simulink model "mixer"  (R2024b)
settings: configuration reference "simulation" (kept outside this file)
values from neighbouring files (symbols this model uses):
  fw_mixers =     [mixer_data.mat]
  mc_mixers =     [mixer_data.mat]
undefined symbols (not defined in the file or in its folder): MC_AIRMODE, MOT_SLEW_MAX, PWM_AUX_DIS1, PWM_AUX_DIS2, PWM_AUX_DIS3, PWM_AUX_DIS4, PWM_AUX_DIS5, PWM_AUX_DIS6, PWM_AUX_DIS7, PWM_AUX_DIS8, PWM_AUX_DISARM, PWM_AUX_FAIL1, PWM_AUX_FAIL2, PWM_AUX_FAIL3, PWM_AUX_FAIL4, PWM_AUX_FAIL5, PWM_AUX_FAIL6, PWM_AUX_FAIL7, PWM_AUX_FAIL8, PWM_AUX_MAX, PWM_AUX_MAX1, PWM_AUX_MAX2, PWM_AUX_MAX3, PWM_AUX_MAX4, PWM_AUX_MAX5, PWM_AUX_MAX6, PWM_AUX_MAX7, PWM_AUX_MAX8, PWM_AUX_MIN, PWM_AUX_MIN1, PWM_AUX_MIN2, PWM_AUX_MIN3, PWM_AUX_MIN4, PWM_AUX_MIN5, PWM_AUX_MIN6, PWM_AUX_REV1, PWM_AUX_REV2, PWM_AUX_REV3, PWM_AUX_REV4, PWM_AUX_REV5, PWM_AUX_REV6, PWM_AUX_REV7, PWM_AUX_REV8, PWM_AUX_TRIM1, PWM_AUX_TRIM2, PWM_AUX_TRIM3, PWM_AUX_TRIM4, PWM_AUX_TRIM5, PWM_AUX_TRIM6, PWM_AUX_TRIM7, PWM_AUX_TRIM8, PWM_MAIN_DIS1, PWM_MAIN_DIS2, PWM_MAIN_DIS3, PWM_MAIN_DIS4, PWM_MAIN_DIS5, PWM_MAIN_DIS6, PWM_MAIN_DIS7, PWM_MAIN_DIS8, PWM_MAIN_DISARM ... (+43)
libraries: simulink x4
settings Model: DataDictionary=nextpilot_datadict.sldd  Creator=CETCA  LastModifiedBy=93114
settings ConfigSetRef: SourceName=simulation

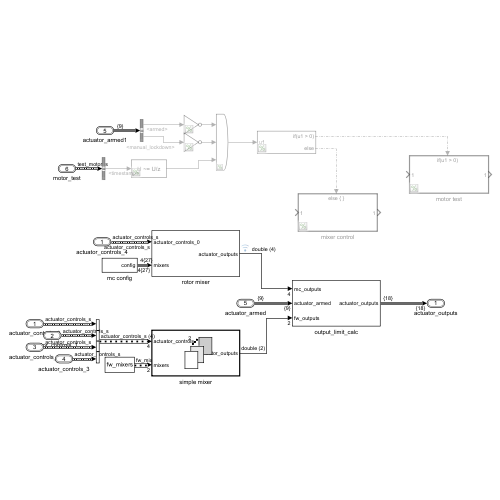
[thumbnail: Simulink's stored preview of the top-level diagram]
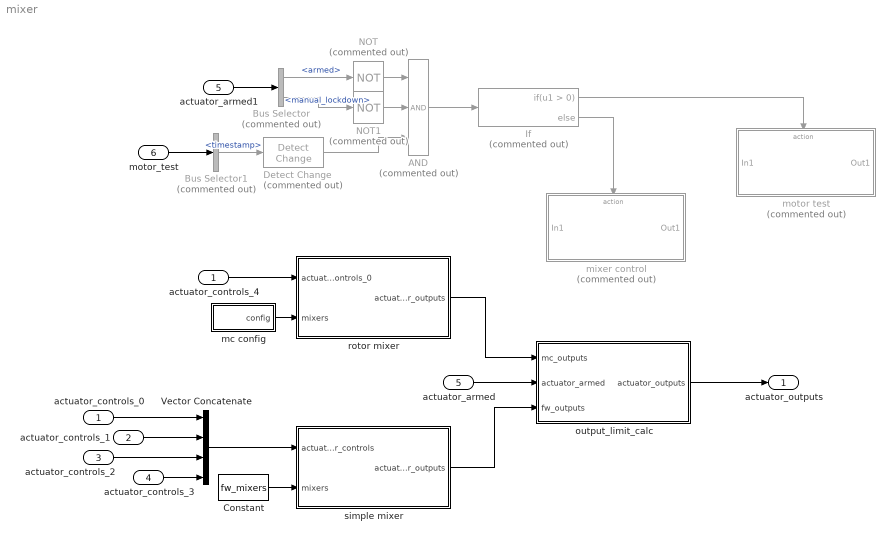
== system mixer ==
  actuator_controls_0 : Inport  OutDataTypeStr=Bus: actuator_controls_s  BusOutputAsStruct=on
  actuator_controls_1 : Inport  Port=2  OutDataTypeStr=Bus: actuator_controls_s  BusOutputAsStruct=on
  actuator_controls_2 : Inport  Port=3  OutDataTypeStr=Bus: actuator_controls_s  BusOutputAsStruct=on
  actuator_controls_3 : Inport  Port=4  OutDataTypeStr=Bus: actuator_controls_s  BusOutputAsStruct=on
  actuator_armed : Inport  Port=5  OutDataTypeStr=Bus: actuator_armed_s
  motor_test : Inport  Port=6  OutDataTypeStr=Bus: test_motor_s  BusOutputAsStruct=on
  AND : Logic  Commented=on  Inputs=3  IconShape=distinctive  AllPortsSameDT=off  OutDataTypeStr=boolean
  Bus Selector : BusSelector  Commented=on  OutputSignals=armed,manual_lockdown
  Bus Selector1 : BusSelector  Commented=on  OutputSignals=timestamp
  Constant : Constant  Value=fw_mixers  OutDataTypeStr=Bus: fw_mixer_s
  Detect Change : simulink/Logic and Bit Operations/Detect Change  Commented=on  vinit=0  OutDataTypeStr=boolean
  If : If  Commented=on
  NOT : Logic  Commented=on  Operator=NOT  IconShape=distinctive  AllPortsSameDT=off  OutDataTypeStr=boolean
  NOT1 : Logic  Commented=on  Operator=NOT  IconShape=distinctive  AllPortsSameDT=off  OutDataTypeStr=boolean
  Vector Concatenate : Concatenate  NumInputs=4
  actuator_armed1 : InportShadow  Port=5  OutDataTypeStr=Bus: actuator_armed_s
  actuator_controls_4 : InportShadow  OutDataTypeStr=Bus: actuator_controls_s  BusOutputAsStruct=on
  mc config : Subsystem
  mixer control : Subsystem  Commented=on  TreatAsAtomicUnit=on
  motor test : Subsystem  Commented=on  TreatAsAtomicUnit=on
  output_limit_calc : Subsystem
  rotor mixer : Subsystem
  simple mixer : Subsystem  TreatAsAtomicUnit=on
  actuator_outputs : Outport  OutDataTypeStr=Bus: actuator_outputs_s
  wires:
  Constant/1 -> simple mixer/2(mixers)
  actuator_controls_0/1 -> Vector Concatenate/1
  actuator_controls_1/1 -> Vector Concatenate/2
  actuator_controls_2/1 -> Vector Concatenate/3
  actuator_controls_3/1 -> Vector Concatenate/4
  Vector Concatenate/1 -> simple mixer/1(actuator_controls)
  rotor mixer/1(actuator_outputs) -> output_limit_calc/1(mc_outputs)
  simple mixer/1(actuator_outputs) -> output_limit_calc/3(fw_outputs)
  output_limit_calc/1(actuator_outputs) -> actuator_outputs/1
  actuator_armed/1 -> output_limit_calc/2(actuator_armed)
  actuator_armed1/1 -> Bus Selector/1
  Bus Selector/1 -> NOT/1  "<armed>"
  Bus Selector/2 -> NOT1/1  "<manual_lockdown>"
  NOT1/1 -> AND/2
  NOT/1 -> AND/1
  AND/1 -> If/1
  motor_test/1 -> Bus Selector1/1
  Bus Selector1/1 -> Detect Change/1  "<timestamp>"
  Detect Change/1 -> AND/3
  If/1 -> motor test/Action
  If/2 -> mixer control/Action
  mc config/1(config) -> rotor mixer/2(mixers)
  actuator_controls_4/1 -> rotor mixer/1(actuator_controls_0)

== system mixer/mc config ==
  Constant : Constant  Value=mc_mixers.type
  Constant1 : Constant  Value=mc_mixers.slew_rate
  Constant2 : Constant  Value=mc_mixers.output_scale
  Constant3 : Constant  Value=mc_mixers.control_scale
  Bus Element Out : Outport  PortName=config  Element=type
  Bus Element Out1 : Outport  PortName=config  Element=slew_rate
  Bus Element Out2 : Outport  PortName=config  Element=output_scale
  Bus Element Out3 : Outport  PortName=config  Element=control_scale
  wires:
  Constant/1 -> Bus Element Out/1
  Constant1/1 -> Bus Element Out1/1
  Constant2/1 -> Bus Element Out2/1
  Constant3/1 -> Bus Element Out3/1

== system mixer/mixer control ==
  In1 : Inport
  Action Port : ActionPort  ActionPortLabel=else
  Out1 : Outport
  wires:
  In1/1 -> Out1/1

== system mixer/motor test ==
  In1 : Inport
  Action Port : ActionPort  ActionPortLabel=if(u1 > 0)
  Out1 : Outport
  wires:
  In1/1 -> Out1/1

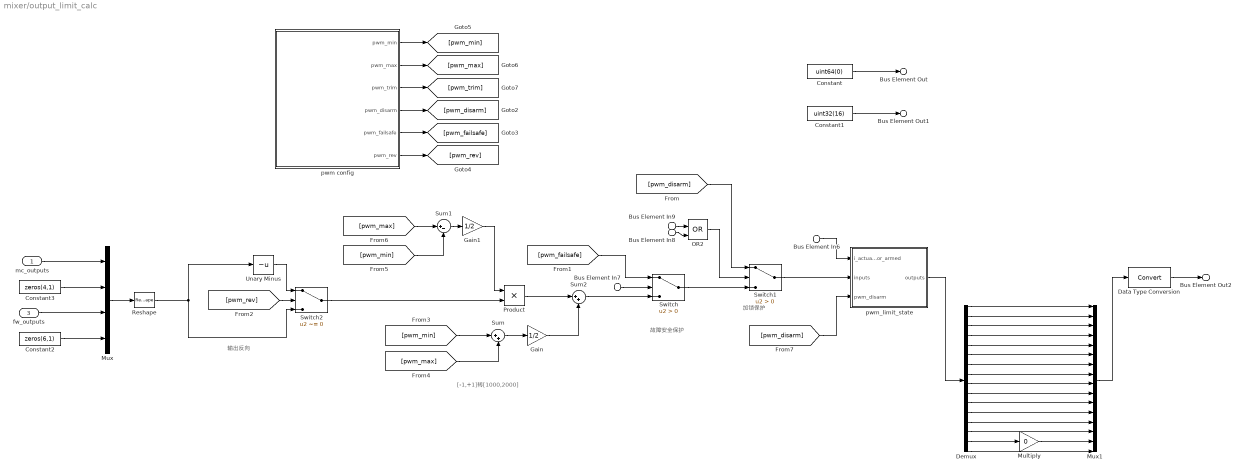
== system mixer/output_limit_calc ==
  note: 故障安全保护
  note: [-1,+1]转[1000,2000]
  note: 输出反向
  note: 加锁保护
  mc_outputs : Inport
  Bus Element In6 : Inport  Port=2  PortName=actuator_armed
  Bus Element In8 : Inport  Port=2  PortName=actuator_armed  Element=lockdown
  Bus Element In7 : Inport  Port=2  PortName=actuator_armed  Element=force_failsafe
  Bus Element In9 : Inport  Port=2  PortName=actuator_armed  Element=manual_lockdown
  fw_outputs : Inport  Port=3
  Constant : Constant  Value=uint64(0)
  Constant1 : Constant  Value=uint32(16)
  Constant2 : Constant  Value=zeros(6,1)
  Constant3 : Constant  Value=zeros(4,1)
  Data Type Conversion : DataTypeConversion  SaturateOnIntegerOverflow=off  RndMeth=Floor
  Demux : Demux  Outputs=16
  Gain : Gain  Gain=1/2
  Gain1 : Gain  Gain=1/2
  Multiply : Gain  Gain=0
  Mux : Mux
  Mux1 : Mux  Inputs=16
  OR2 : Logic  Operator=OR  IconShape=distinctive  AllPortsSameDT=off  OutDataTypeStr=boolean
  Product : Product
  Reshape : Reshape
  Sum : Sum  Inputs=|++
  Sum1 : Sum  Inputs=|+-
  Sum2 : Sum  Inputs=|++
  Switch : Switch  Criteria=u2 > Threshold  SaturateOnIntegerOverflow=off  InputSameDT=off
  Switch1 : Switch  Criteria=u2 > Threshold  SaturateOnIntegerOverflow=off  InputSameDT=off
  Switch2 : Switch  Criteria=u2 ~= 0  SaturateOnIntegerOverflow=off  InputSameDT=off
  Unary Minus : UnaryMinus
  pwm config : Subsystem
  pwm_limit_state : Stateflow chart  TreatAsAtomicUnit=on
  Bus Element Out : Outport  PortName=actuator_outputs  Element=timestamp
  Bus Element Out1 : Outport  PortName=actuator_outputs  Element=noutputs
  Bus Element Out2 : Outport  PortName=actuator_outputs  Element=output
  wires:
  Constant/1 -> Bus Element Out/1
  Constant1/1 -> Bus Element Out1/1
  mc_outputs/1 -> Mux/1
  fw_outputs/1 -> Mux/3
  Constant2/1 -> Mux/4
  Mux/1 -> Reshape/1
  Reshape/1 -> Unary Minus/1, Switch2/3
  Bus Element In6/1 -> pwm_limit_state/1(i_actuator_armed)
  Bus Element In7/1 -> Switch/2
  Switch/1 -> Switch1/3
  Bus Element In9/1 -> OR2/1
  Bus Element In8/1 -> OR2/2
  OR2/1 -> Switch1/2
  Switch1/1 -> pwm_limit_state/2(inputs)
  Data Type Conversion/1 -> Bus Element Out2/1
  pwm config/4(pwm_disarm) -> [pwm_disarm]
  pwm config/5(pwm_failsafe) -> [pwm_failsafe]
  [pwm_disarm] -> Switch1/1
  [pwm_failsafe] -> Switch/1
  pwm config/6(pwm_rev) -> [pwm_rev]
  [pwm_rev] -> Switch2/2
  Unary Minus/1 -> Switch2/1
  pwm config/1(pwm_min) -> [pwm_min]
  pwm config/2(pwm_max) -> [pwm_max]
  [pwm_min] -> Sum/1
  [pwm_max] -> Sum/2
  Sum/1 -> Gain/1
  [pwm_max] -> Sum1/1
  [pwm_min] -> Sum1/2
  Sum1/1 -> Gain1/1
  Gain1/1 -> Product/1
  Switch2/1 -> Product/2
  Product/1 -> Sum2/1
  Gain/1 -> Sum2/2
  Sum2/1 -> Switch/3
  pwm config/3(pwm_trim) -> [pwm_trim]
  pwm_limit_state/1(outputs) -> Demux/1
  [pwm_disarm] -> pwm_limit_state/3(pwm_disarm)
  Constant3/1 -> Mux/2
  Demux/7 -> Mux1/7
  Demux/6 -> Mux1/6
  Demux/8 -> Mux1/8
  Demux/5 -> Mux1/5
  Demux/9 -> Mux1/9
  Demux/4 -> Mux1/4
  Demux/10 -> Mux1/10
  Demux/3 -> Mux1/3
  Demux/11 -> Mux1/11
  Demux/2 -> Mux1/2
  Demux/12 -> Mux1/12
  Demux/1 -> Mux1/1
  Demux/13 -> Mux1/13
  Demux/14 -> Mux1/14
  Demux/15 -> Multiply/1
  Demux/16 -> Mux1/16
  Mux1/1 -> Data Type Conversion/1
  Multiply/1 -> Mux1/15

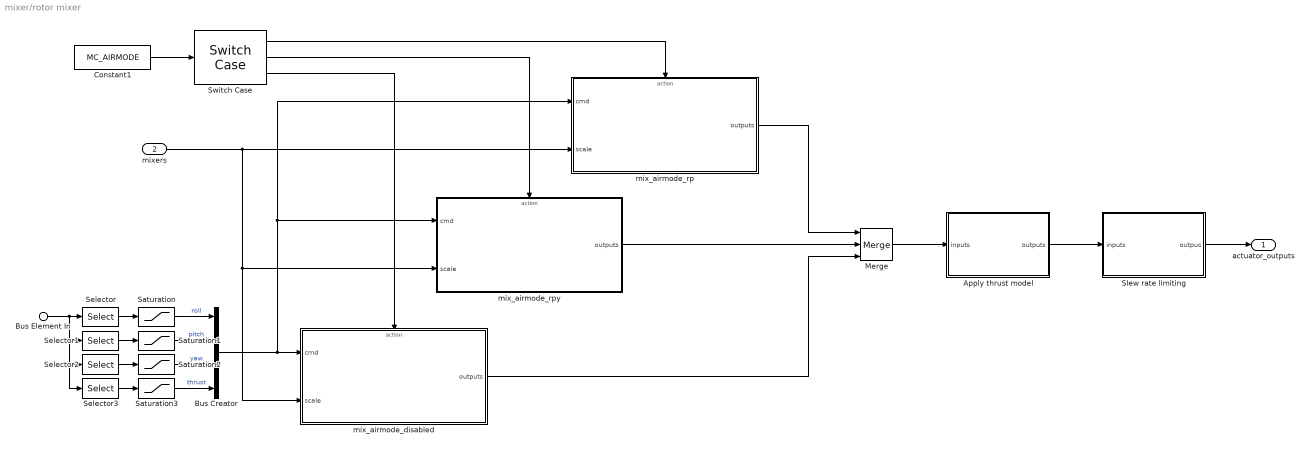
== system mixer/rotor mixer ==
  Bus Element In : Inport  PortName=actuator_controls_0  Element=control
  mixers : Inport  Port=2
  Apply thrust model : Subsystem
  Bus Creator : BusCreator  Inputs=4
  Constant1 : Constant  Value=MC_AIRMODE
  Merge : Merge  Inputs=3
  Saturation : Saturate  UpperLimit=1  LowerLimit=-1
  Saturation1 : Saturate  UpperLimit=1  LowerLimit=-1
  Saturation2 : Saturate  UpperLimit=1  LowerLimit=-1
  Saturation3 : Saturate  UpperLimit=1  LowerLimit=0
  Selector : Selector  InputPortWidth=8  IndexOptions=Index vector (dialog)  Indices=1  OutputSizes=1
  Selector1 : Selector  InputPortWidth=8  IndexOptions=Index vector (dialog)  Indices=2  OutputSizes=1
  Selector2 : Selector  InputPortWidth=8  IndexOptions=Index vector (dialog)  Indices=3  OutputSizes=1
  Selector3 : Selector  InputPortWidth=8  IndexOptions=Index vector (dialog)  Indices=4  OutputSizes=1
  Slew rate limiting : Subsystem
  Switch Case : SwitchCase  CaseConditions={1,2}
  mix_airmode_disabled : Subsystem  TreatAsAtomicUnit=on
  mix_airmode_rp : Subsystem  TreatAsAtomicUnit=on
  mix_airmode_rpy : Subsystem  TreatAsAtomicUnit=on
  actuator_outputs : Outport
  wires:
  Bus Element In/1 -> Selector3/1, Selector2/1, Selector1/1, Selector/1
  Selector/1 -> Saturation/1
  Selector1/1 -> Saturation1/1
  Selector2/1 -> Saturation2/1
  Selector3/1 -> Saturation3/1
  Constant1/1 -> Switch Case/1
  Switch Case/1 -> mix_airmode_rp/Action
  Switch Case/2 -> mix_airmode_rpy/Action
  Switch Case/3 -> mix_airmode_disabled/Action
  Saturation2/1 -> Bus Creator/3  "yaw"
  Saturation1/1 -> Bus Creator/2  "pitch"
  Saturation3/1 -> Bus Creator/4  "thrust"
  Saturation/1 -> Bus Creator/1  "roll"
  Bus Creator/1 -> mix_airmode_rp/1(cmd), mix_airmode_rpy/1(cmd), mix_airmode_disabled/1(cmd)
  mixers/1 -> mix_airmode_rp/2(scale), mix_airmode_rpy/2(scale), mix_airmode_disabled/2(scale)
  mix_airmode_rp/1(outputs) -> Merge/1
  mix_airmode_rpy/1(outputs) -> Merge/2
  mix_airmode_disabled/1(outputs) -> Merge/3
  Merge/1 -> Apply thrust model/1(inputs)
  Apply thrust model/1(outputs) -> Slew rate limiting/1(inputs)
  Slew rate limiting/1(outpus) -> actuator_outputs/1

== system mixer/simple mixer ==
  actuator_controls : Inport  OutDataTypeStr=Bus: actuator_controls_s
  mixers : Inport  Port=2  Partition=on  PartitionDimension=1  PartitionWidth=1  PartitionOffset=0
  Bus Selector : BusSelector  OutputSignals=control_scale
  Bus Selector1 : BusSelector  OutputSignals=output_scale
  Demux : Demux  Outputs=5
  For Each : ForEach  DisableCoverage=on
  Sum : Sum  Inputs=1
  control scale : Subsystem
  output scale : Subsystem
  actuator_outputs : Outport  ConcatenationDimension=1
  wires:
  mixers/1 -> Bus Selector1/1, Bus Selector/1
  actuator_controls/1 -> control scale/1(actuator_controls)
  Bus Selector/1 -> control scale/2(control_scale)  "<control_scale>"
  Sum/1 -> output scale/1(x)
  Demux/2 -> output scale/3(pos_scale)
  Demux/4 -> output scale/5(min)
  Demux/5 -> output scale/6(max)
  Demux/3 -> output scale/4(offset)
  Demux/1 -> output scale/2(neg_scale)
  control scale/1(actuator_outputs) -> Sum/1
  Bus Selector1/1 -> Demux/1  "<output_scale>"
  output scale/1(y) -> actuator_outputs/1

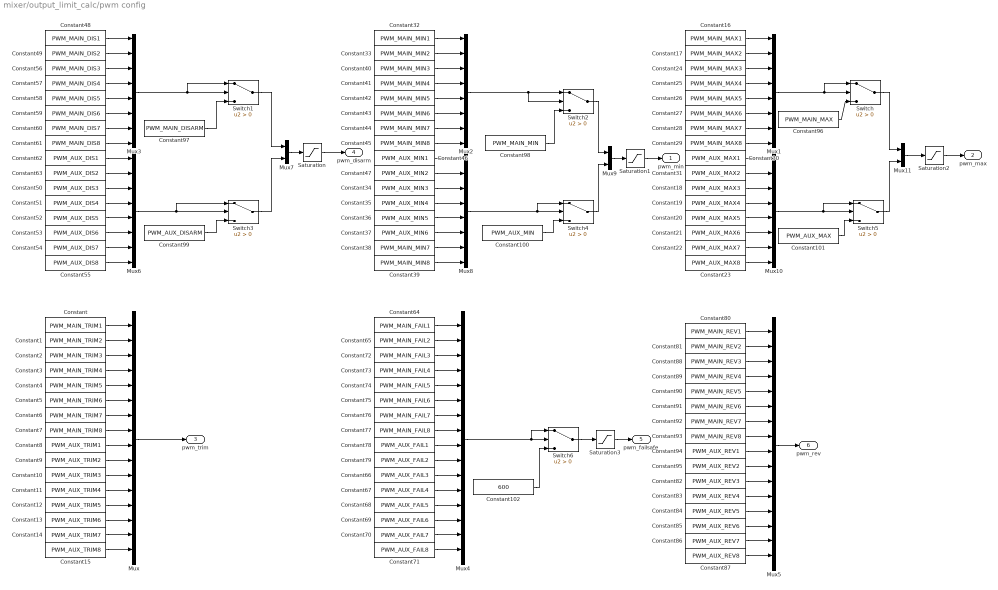
== system mixer/output_limit_calc/pwm config ==
  Constant : Constant  Value=PWM_MAIN_TRIM1
  Constant1 : Constant  Value=PWM_MAIN_TRIM2
  Constant10 : Constant  Value=PWM_AUX_TRIM3
  Constant100 : Constant  Value=PWM_AUX_MIN
  Constant101 : Constant  Value=PWM_AUX_MAX
  Constant102 : Constant  Value=600  OutDataTypeStr=int32
  Constant11 : Constant  Value=PWM_AUX_TRIM4
  Constant12 : Constant  Value=PWM_AUX_TRIM5
  Constant13 : Constant  Value=PWM_AUX_TRIM6
  Constant14 : Constant  Value=PWM_AUX_TRIM7
  Constant15 : Constant  Value=PWM_AUX_TRIM8
  Constant16 : Constant  Value=PWM_MAIN_MAX1
  Constant17 : Constant  Value=PWM_MAIN_MAX2
  Constant18 : Constant  Value=PWM_AUX_MAX3
  Constant19 : Constant  Value=PWM_AUX_MAX4
  Constant2 : Constant  Value=PWM_MAIN_TRIM3
  Constant20 : Constant  Value=PWM_AUX_MAX5
  Constant21 : Constant  Value=PWM_AUX_MAX6
  Constant22 : Constant  Value=PWM_AUX_MAX7
  Constant23 : Constant  Value=PWM_AUX_MAX8
  Constant24 : Constant  Value=PWM_MAIN_MAX3
  Constant25 : Constant  Value=PWM_MAIN_MAX4
  Constant26 : Constant  Value=PWM_MAIN_MAX5
  Constant27 : Constant  Value=PWM_MAIN_MAX6
  Constant28 : Constant  Value=PWM_MAIN_MAX7
  Constant29 : Constant  Value=PWM_MAIN_MAX8
  Constant3 : Constant  Value=PWM_MAIN_TRIM4
  Constant30 : Constant  Value=PWM_AUX_MAX1
  Constant31 : Constant  Value=PWM_AUX_MAX2
  Constant32 : Constant  Value=PWM_MAIN_MIN1
  Constant33 : Constant  Value=PWM_MAIN_MIN2
  Constant34 : Constant  Value=PWM_AUX_MIN3
  Constant35 : Constant  Value=PWM_AUX_MIN4
  Constant36 : Constant  Value=PWM_AUX_MIN5
  Constant37 : Constant  Value=PWM_AUX_MIN6
  Constant38 : Constant  Value=PWM_MAIN_MIN7
  Constant39 : Constant  Value=PWM_MAIN_MIN8
  Constant4 : Constant  Value=PWM_MAIN_TRIM5
  Constant40 : Constant  Value=PWM_MAIN_MIN3
  Constant41 : Constant  Value=PWM_MAIN_MIN4
  Constant42 : Constant  Value=PWM_MAIN_MIN5
  Constant43 : Constant  Value=PWM_MAIN_MIN6
  Constant44 : Constant  Value=PWM_MAIN_MIN7
  Constant45 : Constant  Value=PWM_MAIN_MIN8
  Constant46 : Constant  Value=PWM_AUX_MIN1
  Constant47 : Constant  Value=PWM_AUX_MIN2
  Constant48 : Constant  Value=PWM_MAIN_DIS1
  Constant49 : Constant  Value=PWM_MAIN_DIS2
  Constant5 : Constant  Value=PWM_MAIN_TRIM6
  Constant50 : Constant  Value=PWM_AUX_DIS3
  Constant51 : Constant  Value=PWM_AUX_DIS4
  Constant52 : Constant  Value=PWM_AUX_DIS5
  Constant53 : Constant  Value=PWM_AUX_DIS6
  Constant54 : Constant  Value=PWM_AUX_DIS7
  Constant55 : Constant  Value=PWM_AUX_DIS8
  Constant56 : Constant  Value=PWM_MAIN_DIS3
  Constant57 : Constant  Value=PWM_MAIN_DIS4
  Constant58 : Constant  Value=PWM_MAIN_DIS5
  Constant59 : Constant  Value=PWM_MAIN_DIS6
  Constant6 : Constant  Value=PWM_MAIN_TRIM7
  Constant60 : Constant  Value=PWM_MAIN_DIS7
  Constant61 : Constant  Value=PWM_MAIN_DIS8
  Constant62 : Constant  Value=PWM_AUX_DIS1
  Constant63 : Constant  Value=PWM_AUX_DIS2
  Constant64 : Constant  Value=PWM_MAIN_FAIL1
  Constant65 : Constant  Value=PWM_MAIN_FAIL2
  Constant66 : Constant  Value=PWM_AUX_FAIL3
  Constant67 : Constant  Value=PWM_AUX_FAIL4
  Constant68 : Constant  Value=PWM_AUX_FAIL5
  Constant69 : Constant  Value=PWM_AUX_FAIL6
  Constant7 : Constant  Value=PWM_MAIN_TRIM8
  Constant70 : Constant  Value=PWM_AUX_FAIL7
  Constant71 : Constant  Value=PWM_AUX_FAIL8
  Constant72 : Constant  Value=PWM_MAIN_FAIL3
  Constant73 : Constant  Value=PWM_MAIN_FAIL4
  Constant74 : Constant  Value=PWM_MAIN_FAIL5
  Constant75 : Constant  Value=PWM_MAIN_FAIL6
  Constant76 : Constant  Value=PWM_MAIN_FAIL7
  Constant77 : Constant  Value=PWM_MAIN_FAIL8
  Constant78 : Constant  Value=PWM_AUX_FAIL1
  Constant79 : Constant  Value=PWM_AUX_FAIL2
  Constant8 : Constant  Value=PWM_AUX_TRIM1
  Constant80 : Constant  Value=PWM_MAIN_REV1
  Constant81 : Constant  Value=PWM_MAIN_REV2
  Constant82 : Constant  Value=PWM_AUX_REV3
  Constant83 : Constant  Value=PWM_AUX_REV4
  Constant84 : Constant  Value=PWM_AUX_REV5
  Constant85 : Constant  Value=PWM_AUX_REV6
  Constant86 : Constant  Value=PWM_AUX_REV7
  Constant87 : Constant  Value=PWM_AUX_REV8
  Constant88 : Constant  Value=PWM_MAIN_REV3
  Constant89 : Constant  Value=PWM_MAIN_REV4
  Constant9 : Constant  Value=PWM_AUX_TRIM2
  Constant90 : Constant  Value=PWM_MAIN_REV5
  Constant91 : Constant  Value=PWM_MAIN_REV6
  Constant92 : Constant  Value=PWM_MAIN_REV7
  Constant93 : Constant  Value=PWM_MAIN_REV8
  Constant94 : Constant  Value=PWM_AUX_REV1
  Constant95 : Constant  Value=PWM_AUX_REV2
  Constant96 : Constant  Value=PWM_MAIN_MAX
  Constant97 : Constant  Value=PWM_MAIN_DISARM
  Constant98 : Constant  Value=PWM_MAIN_MIN
  Constant99 : Constant  Value=PWM_AUX_DISARM
  Mux : Mux  Inputs=16
  Mux{1..3,6,8,10} (6 alike) : Mux  Inputs=8
  Mux11 : Mux  Inputs=2
  Mux4 : Mux  Inputs=16
  Mux5 : Mux  Inputs=16
  Mux7 : Mux  Inputs=2
  Mux9 : Mux  Inputs=2
  Saturation : Saturate  UpperLimit=2500  LowerLimit=0
  Saturation1 : Saturate  UpperLimit=1600  LowerLimit=90
  Saturation2 : Saturate  UpperLimit=2500  LowerLimit=200
  Saturation3 : Saturate  UpperLimit=2500  LowerLimit=0
  Switch{,1..6} (7 alike) : Switch  Criteria=u2 > Threshold  SaturateOnIntegerOverflow=off  InputSameDT=off
  pwm_min : Outport
  pwm_max : Outport  Port=2
  pwm_trim : Outport  Port=3
  pwm_disarm : Outport  Port=4
  pwm_failsafe : Outport  Port=5
  pwm_rev : Outport  Port=6
  wires:
  Constant1/1 -> Mux/2
  Constant2/1 -> Mux/3
  Constant/1 -> Mux/1
  Constant3/1 -> Mux/4
  Constant4/1 -> Mux/5
  Constant5/1 -> Mux/6
  Constant6/1 -> Mux/7
  Constant7/1 -> Mux/8
  Constant8/1 -> Mux/9
  Constant9/1 -> Mux/10
  Constant10/1 -> Mux/11
  Constant11/1 -> Mux/12
  Constant12/1 -> Mux/13
  Constant13/1 -> Mux/14
  Constant14/1 -> Mux/15
  Constant15/1 -> Mux/16
  Mux/1 -> pwm_trim/1
  Mux1/1 -> Switch/2, Switch/1
  Constant23/1 -> Mux10/8
  Constant22/1 -> Mux10/7
  Constant21/1 -> Mux10/6
  Constant20/1 -> Mux10/5
  Constant19/1 -> Mux10/4
  Constant18/1 -> Mux10/3
  Constant31/1 -> Mux10/2
  Constant30/1 -> Mux10/1
  Constant29/1 -> Mux1/8
  Constant28/1 -> Mux1/7
  Constant27/1 -> Mux1/6
  Constant26/1 -> Mux1/5
  Constant25/1 -> Mux1/4
  Constant16/1 -> Mux1/1
  Constant24/1 -> Mux1/3
  Constant17/1 -> Mux1/2
  Constant33/1 -> Mux2/2
  Constant40/1 -> Mux2/3
  Constant32/1 -> Mux2/1
  Constant41/1 -> Mux2/4
  Constant42/1 -> Mux2/5
  Constant43/1 -> Mux2/6
  Constant44/1 -> Mux2/7
  Constant45/1 -> Mux2/8
  Constant46/1 -> Mux8/1
  Constant47/1 -> Mux8/2
  Constant34/1 -> Mux8/3
  Constant35/1 -> Mux8/4
  Constant36/1 -> Mux8/5
  Constant37/1 -> Mux8/6
  Constant38/1 -> Mux8/7
  Constant39/1 -> Mux8/8
  Mux2/1 -> Switch2/1, Switch2/2
  Mux3/1 -> Switch1/1, Switch1/2
  Constant55/1 -> Mux6/8
  Constant54/1 -> Mux6/7
  Constant53/1 -> Mux6/6
  Constant52/1 -> Mux6/5
  Constant51/1 -> Mux6/4
  Constant50/1 -> Mux6/3
  Constant63/1 -> Mux6/2
  Constant62/1 -> Mux6/1
  Constant61/1 -> Mux3/8
  Constant60/1 -> Mux3/7
  Constant59/1 -> Mux3/6
  Constant58/1 -> Mux3/5
  Constant57/1 -> Mux3/4
  Constant48/1 -> Mux3/1
  Constant56/1 -> Mux3/3
  Constant49/1 -> Mux3/2
  Constant65/1 -> Mux4/2
  Constant72/1 -> Mux4/3
  Constant64/1 -> Mux4/1
  Constant73/1 -> Mux4/4
  Constant74/1 -> Mux4/5
  Constant75/1 -> Mux4/6
  Constant76/1 -> Mux4/7
  Constant77/1 -> Mux4/8
  Constant78/1 -> Mux4/9
  Constant79/1 -> Mux4/10
  Constant66/1 -> Mux4/11
  Constant67/1 -> Mux4/12
  Constant68/1 -> Mux4/13
  Constant69/1 -> Mux4/14
  Constant70/1 -> Mux4/15
  Constant71/1 -> Mux4/16
  Mux5/1 -> pwm_rev/1
  Constant80/1 -> Mux5/1
  Constant81/1 -> Mux5/2
  Constant88/1 -> Mux5/3
  Constant89/1 -> Mux5/4
  Constant90/1 -> Mux5/5
  Constant91/1 -> Mux5/6
  Constant92/1 -> Mux5/7
  Constant93/1 -> Mux5/8
  Constant94/1 -> Mux5/9
  Constant95/1 -> Mux5/10
  Constant82/1 -> Mux5/11
  Constant83/1 -> Mux5/12
  Constant84/1 -> Mux5/13
  Constant85/1 -> Mux5/14
  Constant86/1 -> Mux5/15
  Constant87/1 -> Mux5/16
  Switch/1 -> Mux11/1
  Constant96/1 -> Switch/3
  Constant97/1 -> Switch1/3
  Mux7/1 -> Saturation/1
  Constant98/1 -> Switch2/3
  Switch2/1 -> Mux9/1
  Mux6/1 -> Switch3/1, Switch3/2
  Constant99/1 -> Switch3/3
  Switch1/1 -> Mux7/1
  Switch3/1 -> Mux7/2
  Mux8/1 -> Switch4/1, Switch4/2
  Constant100/1 -> Switch4/3
  Switch4/1 -> Mux9/2
  Mux9/1 -> Saturation1/1
  Mux10/1 -> Switch5/1, Switch5/2
  Constant101/1 -> Switch5/3
  Switch5/1 -> Mux11/2
  Mux11/1 -> Saturation2/1
  Mux4/1 -> Switch6/1, Switch6/2
  Constant102/1 -> Switch6/3
  Switch6/1 -> Saturation3/1
  Saturation/1 -> pwm_disarm/1
  Saturation1/1 -> pwm_min/1
  Saturation2/1 -> pwm_max/1
  Saturation3/1 -> pwm_failsafe/1

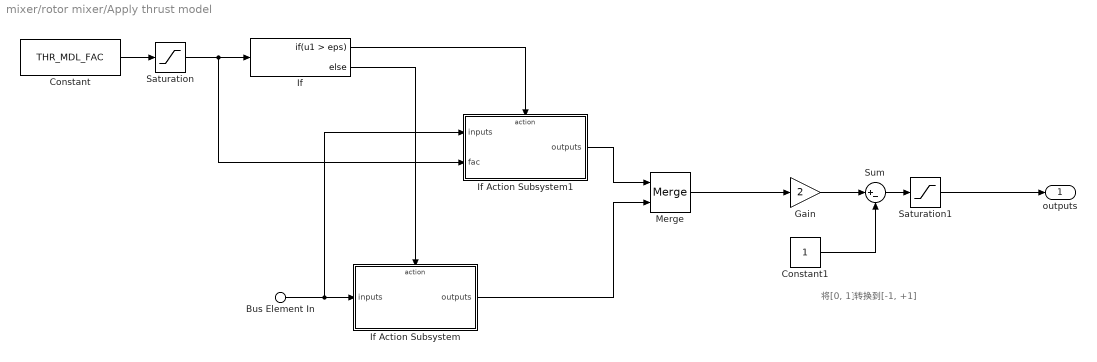
== system mixer/rotor mixer/Apply thrust model ==
  note: 将[0, 1]转换到[-1, +1]
  Bus Element In : Inport  PortName=inputs  Element=outputs
  Constant : Constant  Value=THR_MDL_FAC
  Constant1 : Constant
  Gain : Gain  Gain=2
  If : If  IfExpression=u1 > eps
  If Action Subsystem : Subsystem  TreatAsAtomicUnit=on
  If Action Subsystem1 : Subsystem  TreatAsAtomicUnit=on
  Merge : Merge
  Saturation : Saturate  UpperLimit=1  LowerLimit=0
  Saturation1 : Saturate  UpperLimit=1  LowerLimit=-1
  Sum : Sum  Inputs=|+-
  outputs : Outport
  wires:
  Merge/1 -> Gain/1
  Constant/1 -> Saturation/1
  Gain/1 -> Sum/1
  Sum/1 -> Saturation1/1
  Constant1/1 -> Sum/2
  Saturation1/1 -> outputs/1
  Saturation/1 -> If Action Subsystem1/2(fac), If/1
  Bus Element In/1 -> If Action Subsystem1/1(inputs), If Action Subsystem/1(inputs)
  If Action Subsystem/1(outputs) -> Merge/2
  If/2 -> If Action Subsystem/Action
  If/1 -> If Action Subsystem1/Action
  If Action Subsystem1/1(outputs) -> Merge/1

== system mixer/rotor mixer/Slew rate limiting ==
  note: % /**
      | % * Minimum motor rise time (slew rate limit).
      | % *
      | % * Minimum time allowed for the motor input signal to pass through
      | % * a range of 1000 PWM units. A value x means that the motor signal
      | % * can only go from 1000 to 2000 PWM in maximum x seconds.
      | % *
      | % * Zero means that slew rate limiting is disabled.
      | % *
      | % * @min 0.0
      | % * @unit s/(1000*PWM)
      | % * @group PWM Outputs
      | % */
  inputs : Inport
  Constant9 : Constant  Value=MOT_SLEW_MAX
  If : If  IfExpression=u1 > eps
  Merge : Merge
  Switch Case Action Subsystem : Subsystem  TreatAsAtomicUnit=on
  Switch Case Action Subsystem1 : Subsystem  TreatAsAtomicUnit=on
  outpus : Outport
  wires:
  Merge/1 -> outpus/1
  inputs/1 -> Switch Case Action Subsystem1/1(inputs), Switch Case Action Subsystem/1(inputs)
  Constant9/1 -> Switch Case Action Subsystem1/2(slew), If/1
  Switch Case Action Subsystem/1(outputs) -> Merge/2
  Switch Case Action Subsystem1/1(outputs) -> Merge/1
  If/2 -> Switch Case Action Subsystem/Action
  If/1 -> Switch Case Action Subsystem1/Action

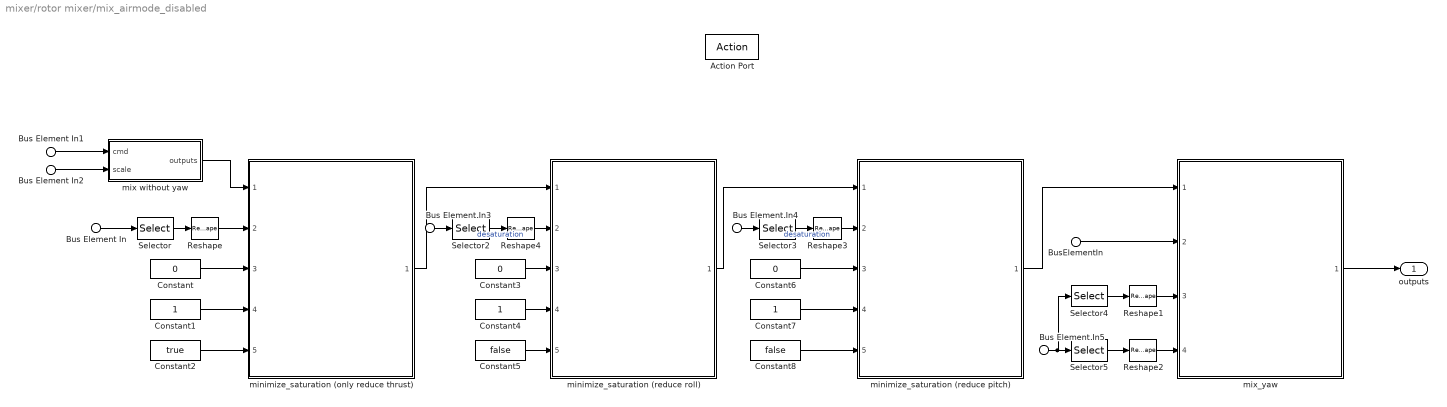
== system mixer/rotor mixer/mix_airmode_disabled ==
  Bus Element In1 : Inport  PortName=cmd
  BusElementIn : Inport  PortName=cmd  Element=yaw
  Bus Element In2 : Inport  Port=2  PortName=scale
  Bus Element In{,3..5} (4 alike) : Inport  Port=2  PortName=scale  Element=control_scale
  Action Port : ActionPort  ActionPortLabel=default:
  Constant : Constant  Value=0
  Constant1 : Constant
  Constant2 : Constant  Value=true
  Constant3 : Constant  Value=0
  Constant4 : Constant
  Constant5 : Constant  Value=false
  Constant6 : Constant  Value=0
  Constant7 : Constant
  Constant8 : Constant  Value=false
  Reshape{,1..4} (5 alike) : Reshape
  Selector : Selector  NumberOfDimensions=2  InputPortWidth=3  IndexOptions=Select all,Index vector (dialog)  Indices=[1 3],4  OutputSizes=1,1
  Selector2 : Selector  NumberOfDimensions=2  InputPortWidth=3  IndexOptions=Select all,Index vector (dialog)  Indices=[1 3],1  OutputSizes=1,1
  Selector3 : Selector  NumberOfDimensions=2  InputPortWidth=3  IndexOptions=Select all,Index vector (dialog)  Indices=[1 3],2  OutputSizes=1,1
  Selector4 : Selector  NumberOfDimensions=2  InputPortWidth=3  IndexOptions=Select all,Index vector (dialog)  Indices=[1 3],3  OutputSizes=1,1
  Selector5 : Selector  NumberOfDimensions=2  InputPortWidth=3  IndexOptions=Select all,Index vector (dialog)  Indices=[1 3],4  OutputSizes=1,1
  minimize_saturation (only reduce thrust) : Subsystem  ReferencedSubsystem=subref_minimize_saturation
  minimize_saturation (reduce pitch) : Subsystem  ReferencedSubsystem=subref_minimize_saturation
  minimize_saturation (reduce roll) : Subsystem  ReferencedSubsystem=subref_minimize_saturation
  mix without yaw : Subsystem
  mix_yaw : Subsystem  ReferencedSubsystem=subref_mix_yaw
  outputs : Outport
  wires:
  Bus Element In/1 -> Selector/1
  Selector/1 -> Reshape/1
  Constant/1 -> minimize_saturation (only reduce thrust)/3
  Constant1/1 -> minimize_saturation (only reduce thrust)/4
  Constant2/1 -> minimize_saturation (only reduce thrust)/5
  Bus Element In3/1 -> Selector2/1
  Selector2/1 -> Reshape4/1  "desaturation"
  Constant3/1 -> minimize_saturation (reduce roll)/3
  Constant4/1 -> minimize_saturation (reduce roll)/4
  Constant5/1 -> minimize_saturation (reduce roll)/5
  minimize_saturation (only reduce thrust)/1 -> minimize_saturation (reduce roll)/1
  minimize_saturation (reduce roll)/1 -> minimize_saturation (reduce pitch)/1
  Bus Element In4/1 -> Selector3/1
  Selector3/1 -> Reshape3/1  "desaturation"
  Constant6/1 -> minimize_saturation (reduce pitch)/3
  Constant7/1 -> minimize_saturation (reduce pitch)/4
  Constant8/1 -> minimize_saturation (reduce pitch)/5
  BusElementIn/1 -> mix_yaw/2
  Bus Element In5/1 -> Selector4/1, Selector5/1
  Selector4/1 -> Reshape1/1
  minimize_saturation (reduce pitch)/1 -> mix_yaw/1
  Selector5/1 -> Reshape2/1
  mix_yaw/1 -> outputs/1
  Bus Element In2/1 -> mix without yaw/2(scale)
  Bus Element In1/1 -> mix without yaw/1(cmd)
  mix without yaw/1(outputs) -> minimize_saturation (only reduce thrust)/1
  Reshape/1 -> minimize_saturation (only reduce thrust)/2
  Reshape1/1 -> mix_yaw/3
  Reshape2/1 -> mix_yaw/4
  Reshape3/1 -> minimize_saturation (reduce pitch)/2
  Reshape4/1 -> minimize_saturation (reduce roll)/2

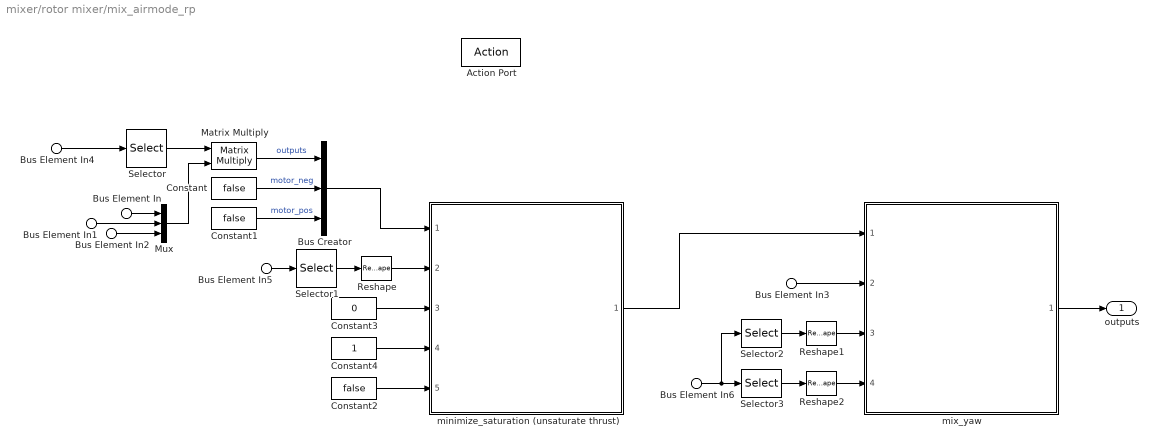
== system mixer/rotor mixer/mix_airmode_rp ==
  Bus Element In : Inport  PortName=cmd  Element=roll
  Bus Element In1 : Inport  PortName=cmd  Element=pitch
  Bus Element In2 : Inport  PortName=cmd  Element=thrust
  Bus Element In3 : Inport  PortName=cmd  Element=yaw
  Bus Element In4 : Inport  Port=2  PortName=scale  Element=control_scale
  Bus Element In5 : Inport  Port=2  PortName=scale  Element=control_scale
  Bus Element In6 : Inport  Port=2  PortName=scale  Element=control_scale
  Action Port : ActionPort  ActionPortLabel=case [ 1 ]:
  Bus Creator : BusCreator  Inputs=3
  Constant : Constant  Value=false
  Constant1 : Constant  Value=false
  Constant2 : Constant  Value=false
  Constant3 : Constant  Value=0
  Constant4 : Constant
  Matrix Multiply : Product  Multiplication=Matrix(*)
  Mux : Mux  Inputs=3
  Reshape : Reshape
  Reshape1 : Reshape
  Reshape2 : Reshape
  Selector : Selector  NumberOfDimensions=2  InputPortWidth=3  IndexOptions=Select all,Index vector (dialog)  Indices=[1 3],[1 2 4]  OutputSizes=1,1
  Selector1 : Selector  NumberOfDimensions=2  InputPortWidth=3  IndexOptions=Select all,Index vector (dialog)  Indices=[1 3],4  OutputSizes=1,1
  Selector2 : Selector  NumberOfDimensions=2  InputPortWidth=3  IndexOptions=Select all,Index vector (dialog)  Indices=[1 3],3  OutputSizes=1,1
  Selector3 : Selector  NumberOfDimensions=2  InputPortWidth=3  IndexOptions=Select all,Index vector (dialog)  Indices=[1 3],4  OutputSizes=1,1
  minimize_saturation (unsaturate thrust) : Subsystem  ReferencedSubsystem=subref_minimize_saturation
  mix_yaw : Subsystem  ReferencedSubsystem=subref_mix_yaw
  outputs : Outport
  wires:
  Bus Element In1/1 -> Mux/2
  Bus Element In2/1 -> Mux/3
  Bus Element In/1 -> Mux/1
  Bus Element In4/1 -> Selector/1
  Selector/1 -> Matrix Multiply/1
  Mux/1 -> Matrix Multiply/2
  Matrix Multiply/1 -> Bus Creator/1  "outputs"
  Constant/1 -> Bus Creator/2  "motor_neg"
  Constant1/1 -> Bus Creator/3  "motor_pos"
  Bus Creator/1 -> minimize_saturation (unsaturate thrust)/1
  Bus Element In5/1 -> Selector1/1
  Selector1/1 -> Reshape/1
  Constant2/1 -> minimize_saturation (unsaturate thrust)/5
  Constant3/1 -> minimize_saturation (unsaturate thrust)/3
  Constant4/1 -> minimize_saturation (unsaturate thrust)/4
  minimize_saturation (unsaturate thrust)/1 -> mix_yaw/1
  Bus Element In3/1 -> mix_yaw/2
  Bus Element In6/1 -> Selector2/1, Selector3/1
  Selector2/1 -> Reshape1/1
  Selector3/1 -> Reshape2/1
  mix_yaw/1 -> outputs/1
  Reshape/1 -> minimize_saturation (unsaturate thrust)/2
  Reshape1/1 -> mix_yaw/3
  Reshape2/1 -> mix_yaw/4

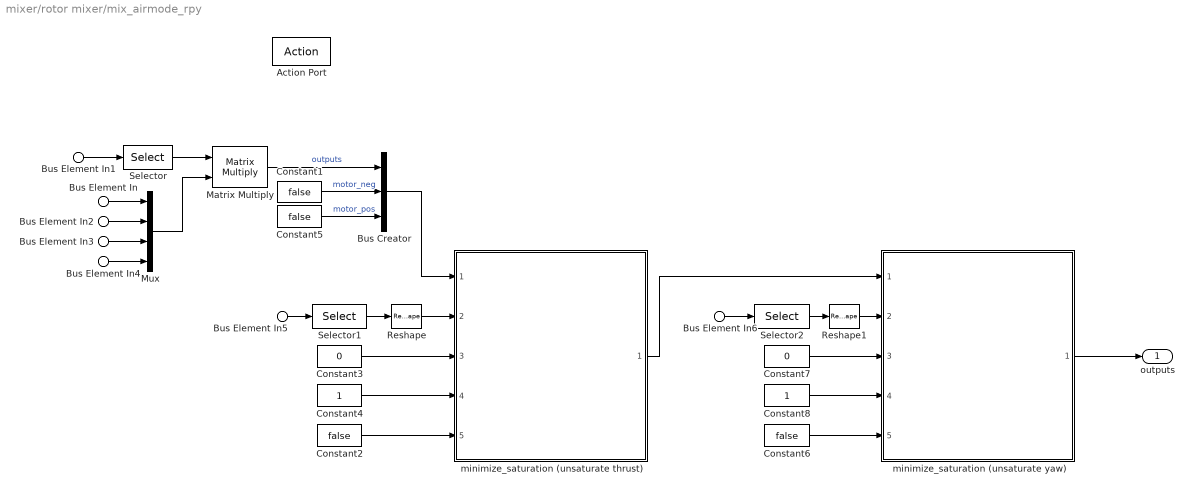
== system mixer/rotor mixer/mix_airmode_rpy ==
  Bus Element In : Inport  PortName=cmd  Element=roll
  Bus Element In2 : Inport  PortName=cmd  Element=pitch
  Bus Element In3 : Inport  PortName=cmd  Element=yaw
  Bus Element In4 : Inport  PortName=cmd  Element=thrust
  Bus Element In1 : Inport  Port=2  PortName=scale  Element=control_scale
  Bus Element In5 : Inport  Port=2  PortName=scale  Element=control_scale
  Bus Element In6 : Inport  Port=2  PortName=scale  Element=control_scale
  Action Port : ActionPort  ActionPortLabel=case [ 2 ]:
  Bus Creator : BusCreator  Inputs=3
  Constant{1..2,5..6} (4 alike) : Constant  Value=false
  Constant3 : Constant  Value=0
  Constant4 : Constant
  Constant7 : Constant  Value=0
  Constant8 : Constant
  Matrix Multiply : Product  Multiplication=Matrix(*)
  Mux : Mux
  Reshape : Reshape
  Reshape1 : Reshape
  Selector : Selector  NumberOfDimensions=2  InputPortWidth=3  IndexOptions=Select all,Index vector (dialog)  Indices=[1 3],[1 2 3 4]  OutputSizes=1,1
  Selector1 : Selector  NumberOfDimensions=2  InputPortWidth=3  IndexOptions=Select all,Index vector (dialog)  Indices=[1 3],4  OutputSizes=1,1
  Selector2 : Selector  NumberOfDimensions=2  InputPortWidth=3  IndexOptions=Select all,Index vector (dialog)  Indices=[1 3],3  OutputSizes=1,1
  minimize_saturation (unsaturate thrust) : Subsystem  ReferencedSubsystem=subref_minimize_saturation
  minimize_saturation (unsaturate yaw) : Subsystem  ReferencedSubsystem=subref_minimize_saturation
  outputs : Outport
  wires:
  Bus Element In2/1 -> Mux/2
  Bus Element In/1 -> Mux/1
  Bus Element In3/1 -> Mux/3
  Bus Element In4/1 -> Mux/4
  Mux/1 -> Matrix Multiply/2
  Bus Element In1/1 -> Selector/1
  Selector/1 -> Matrix Multiply/1
  Bus Element In5/1 -> Selector1/1
  Selector1/1 -> Reshape/1
  Constant3/1 -> minimize_saturation (unsaturate thrust)/3
  Constant4/1 -> minimize_saturation (unsaturate thrust)/4
  Constant2/1 -> minimize_saturation (unsaturate thrust)/5
  Matrix Multiply/1 -> Bus Creator/1  "outputs"
  Constant1/1 -> Bus Creator/2  "motor_neg"
  Bus Creator/1 -> minimize_saturation (unsaturate thrust)/1
  Constant5/1 -> Bus Creator/3  "motor_pos"
  minimize_saturation (unsaturate thrust)/1 -> minimize_saturation (unsaturate yaw)/1
  Selector2/1 -> Reshape1/1
  Bus Element In6/1 -> Selector2/1
  Constant7/1 -> minimize_saturation (unsaturate yaw)/3
  Constant8/1 -> minimize_saturation (unsaturate yaw)/4
  Constant6/1 -> minimize_saturation (unsaturate yaw)/5
  minimize_saturation (unsaturate yaw)/1 -> outputs/1
  Reshape/1 -> minimize_saturation (unsaturate thrust)/2
  Reshape1/1 -> minimize_saturation (unsaturate yaw)/2

== system mixer/simple mixer/control scale ==
  actuator_controls : Inport
  control_scale : Inport  Port=2  Partition=on  PartitionDimension=1  PartitionWidth=1  PartitionOffset=0
  Bus Selector : BusSelector  OutputSignals=control
  Demux : Demux  Outputs=7
  For Each : ForEach  DisableCoverage=on
  Reshape : Reshape
  Selector : Selector  IndexMode=Zero-based  InputPortWidth=4  IndexOptions=Index vector (port)  Indices=[1 3]  OutputSizes=1
  Selector1 : Selector  IndexMode=Zero-based  InputPortWidth=8  IndexOptions=Index vector (port)  Indices=[1 3]  OutputSizes=1
  Subsystem : Subsystem
  actuator_outputs : Outport  ConcatenationDimension=1
  wires:
  Demux/4 -> Subsystem/3(pos_scale)  "pos_scale"
  Subsystem/1(y) -> actuator_outputs/1
  Demux/3 -> Subsystem/2(neg_scale)  "neg_scale"
  Demux/5 -> Subsystem/4(offset)  "offset"
  Selector1/1 -> Subsystem/1(x)
  Demux/1 -> Selector/2  "group"
  Selector/1 -> Bus Selector/1
  Demux/2 -> Selector1/2  "index"
  Demux/6 -> Subsystem/5(min)  "min"
  Demux/7 -> Subsystem/6(max)  "max"
  actuator_controls/1 -> Selector/1
  control_scale/1 -> Reshape/1
  Bus Selector/1 -> Selector1/1  "<control>"
  Reshape/1 -> Demux/1

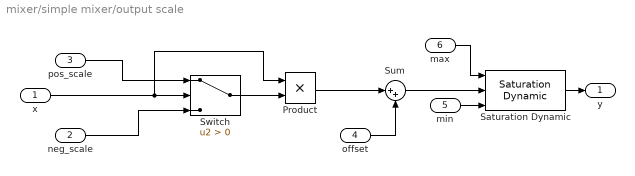
== system mixer/simple mixer/output scale ==
  x : Inport
  neg_scale : Inport  Port=2
  pos_scale : Inport  Port=3
  offset : Inport  Port=4
  min : Inport  Port=5
  max : Inport  Port=6
  Product : Product
  Saturation Dynamic : simulink/Discontinuities/Saturation Dynamic  OutMin=[]  OutMax=[]  OutDataTypeStr=Inherit: Same as second input  OutDataType=fixdt(1, 16)  OutScaling=2^-10  DoSatur=off
  Sum : Sum  Inputs=|++
  Switch : Switch  Criteria=u2 > Threshold  SaturateOnIntegerOverflow=off  InputSameDT=off
  y : Outport
  wires:
  neg_scale/1 -> Switch/3
  max/1 -> Saturation Dynamic/1
  Sum/1 -> Saturation Dynamic/2
  pos_scale/1 -> Switch/1
  Saturation Dynamic/1 -> y/1
  Product/1 -> Sum/1
  Switch/1 -> Product/2
  x/1 -> Switch/2, Product/1
  offset/1 -> Sum/2
  min/1 -> Saturation Dynamic/3

== system mixer/rotor mixer/Apply thrust model/If Action Subsystem ==
  inputs : Inport
  Action Port : ActionPort  ActionPortLabel=else
  outputs : Outport
  wires:
  inputs/1 -> outputs/1

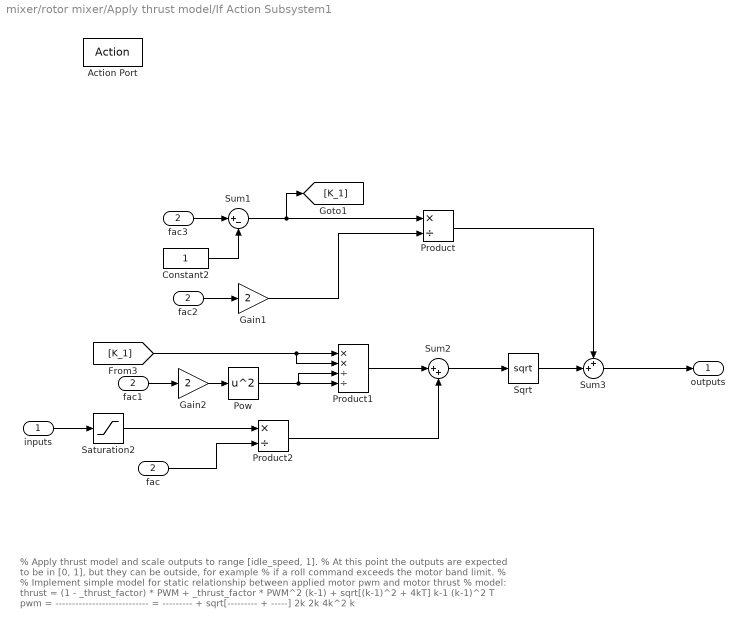
== system mixer/rotor mixer/Apply thrust model/If Action Subsystem1 ==
  note: % Apply thrust model and scale outputs to range [idle_speed, 1].
      | % At this point the outputs are expected to be in [0, 1], but they can be outside, for example
      | % if a roll command exceeds the motor band limit.
      | %
      | % Implement simple model for static relationship between applied motor pwm and motor thrust
      | % model: thrust = (1 - _thrust_factor) * PWM + _thrust_factor * PWM^2
      |
      | (k-1) + sqrt[(k-1)^2 + 4kT] k-1 (k-1)^2 T
      | pwm = ---------------------------- = --------- + sqrt[--------- + -----]
      | 2k 2k 4k^2 k
  inputs : Inport
  fac : Inport  Port=2
  Action Port : ActionPort  ActionPortLabel=if(u1 > eps)
  Constant2 : Constant
  Gain1 : Gain  Gain=2
  Gain2 : Gain  Gain=2
  Pow : Math  Operator=square  SignedPower=on  RndMeth=Zero
  Product : Product  Inputs=*/
  Product1 : Product  Inputs=**//
  Product2 : Product  Inputs=*/
  Saturation2 : Saturate  UpperLimit=inf  LowerLimit=0
  Sqrt : Sqrt
  Sum1 : Sum  Inputs=|+-
  Sum2 : Sum  Inputs=|++
  Sum3 : Sum  Inputs=++|
  fac1 : InportShadow  Port=2
  fac2 : InportShadow  Port=2
  fac3 : InportShadow  Port=2
  outputs : Outport
  wires:
  Gain1/1 -> Product/2
  Constant2/1 -> Sum1/2
  [K_1] -> Product1/2, Product1/1
  Sum3/1 -> outputs/1
  Product1/1 -> Sum2/1
  Product/1 -> Sum3/1
  Saturation2/1 -> Product2/1
  Pow/1 -> Product1/4, Product1/3
  Sum1/1 -> [K_1], Product/1
  fac1/1 -> Gain2/1
  Product2/1 -> Sum2/2
  Sqrt/1 -> Sum3/2
  fac2/1 -> Gain1/1
  fac3/1 -> Sum1/1
  Gain2/1 -> Pow/1
  fac/1 -> Product2/2
  Sum2/1 -> Sqrt/1
  inputs/1 -> Saturation2/1

== system mixer/rotor mixer/Slew rate limiting/Switch Case Action Subsystem ==
  inputs : Inport
  Action Port : ActionPort  ActionPortLabel=else
  outputs : Outport
  wires:
  inputs/1 -> outputs/1

== system mixer/rotor mixer/Slew rate limiting/Switch Case Action Subsystem1 ==
  inputs : Inport
  slew : Inport  Port=2
  Action Port : ActionPort  ActionPortLabel=if(u1 > eps)
  Constant1 : Constant  Value=2
  Product : Product  Inputs=*/
  Rate Limiter Dynamic : simulink/Discontinuities/Rate Limiter Dynamic
  Unary Minus : UnaryMinus
  outputs : Outport
  wires:
  Rate Limiter Dynamic/1 -> outputs/1
  Product/1 -> Unary Minus/1, Rate Limiter Dynamic/1
  inputs/1 -> Rate Limiter Dynamic/2
  Constant1/1 -> Product/1
  Unary Minus/1 -> Rate Limiter Dynamic/3
  slew/1 -> Product/2

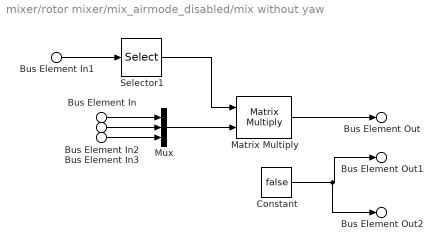
== system mixer/rotor mixer/mix_airmode_disabled/mix without yaw ==
  Bus Element In : Inport  PortName=cmd  Element=roll
  Bus Element In2 : Inport  PortName=cmd  Element=pitch
  Bus Element In3 : Inport  PortName=cmd  Element=thrust
  Bus Element In1 : Inport  Port=2  PortName=scale  Element=control_scale
  Constant : Constant  Value=false
  Matrix Multiply : Product  Multiplication=Matrix(*)
  Mux : Mux  Inputs=3
  Selector1 : Selector  NumberOfDimensions=2  InputPortWidth=3  IndexOptions=Select all,Index vector (dialog)  Indices=[1 3],[1 2 4]  OutputSizes=1,1
  Bus Element Out : Outport  PortName=outputs  Element=outputs
  Bus Element Out1 : Outport  PortName=outputs  Element=motor_neg
  Bus Element Out2 : Outport  PortName=outputs  Element=motor_pos
  wires:
  Bus Element In2/1 -> Mux/2
  Selector1/1 -> Matrix Multiply/1
  Bus Element In3/1 -> Mux/3
  Mux/1 -> Matrix Multiply/2
  Bus Element In/1 -> Mux/1
  Matrix Multiply/1 -> Bus Element Out/1
  Bus Element In1/1 -> Selector1/1
  Constant/1 -> Bus Element Out2/1, Bus Element Out1/1

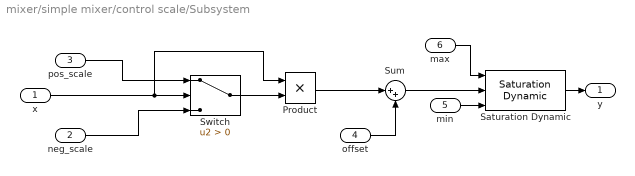
== system mixer/simple mixer/control scale/Subsystem ==
  x : Inport
  neg_scale : Inport  Port=2
  pos_scale : Inport  Port=3
  offset : Inport  Port=4
  min : Inport  Port=5
  max : Inport  Port=6
  Product : Product
  Saturation Dynamic : simulink/Discontinuities/Saturation Dynamic  OutMin=[]  OutMax=[]  OutDataTypeStr=Inherit: Same as second input  OutDataType=fixdt(1, 16)  OutScaling=2^-10  DoSatur=off
  Sum : Sum  Inputs=|++
  Switch : Switch  Criteria=u2 > Threshold  SaturateOnIntegerOverflow=off  InputSameDT=off
  y : Outport
  wires:
  min/1 -> Saturation Dynamic/3
  offset/1 -> Sum/2
  x/1 -> Product/1, Switch/2
  Switch/1 -> Product/2
  Product/1 -> Sum/1
  Saturation Dynamic/1 -> y/1
  pos_scale/1 -> Switch/1
  Sum/1 -> Saturation Dynamic/2
  max/1 -> Saturation Dynamic/1
  neg_scale/1 -> Switch/3

== stateflow chart mixer/output_limit_calc/pwm_limit_state ==
  state pwm_output_limit [parallel]
    en,du:
    throttle_armed   = (i_actuator_armed.armed && ~i_actuator_armed.lockdown) || i_actuator_armed.in_esc_calibration_mode;
    arm_no_throttle = (i_actuator_armed.prearmed && ~i_actuator_armed.armed) || i_actuator_armed.in_esc_calibration_mode;
    settings: executionOrder=1
    state ON
      en,du:
      outputs = inputs;
    state INIT
      en,du:
      outputs(:) = pwm_disarm(:);
    state OFF
      en,du:
      outputs(:) = pwm_disarm(:);
    state RAMP
      en,du:
      outputs = inputs;
    RAMP -> OFF [order 1] : [~throttle_armed]
    (default) -> INIT
    INIT -> OFF : [throttle_armed && after(0.05,sec)]
    OFF -> RAMP : [throttle_armed]
    RAMP -> ON [order 2] : after(0.05,sec)
    ON -> OFF : [~throttle_armed]
  data: i_actuator_armed input; inputs input; outputs output; pwm_disarm input; arm_no_throttle local; throttle_armed local
